simulink model "SetMultipleLedExample"  (R2015a)
settings: Solver=ode3  SolverMode=SingleTasking  StartTime=0.0  StopTime=10.0  RelTol=1e-3
settings Model: ExtModeTrigDuration=2  Creator=kkhoo  LastModifiedBy=kkhoo
settings OptimizationCC: OptimizeModelRefInitCode=on  LifeSpan=1
settings DebuggingCC: UnderspecifiedInitializationDetection=Classic  MergeDetectMultiDrivingBlocksExec=none
settings HardwareCC: ProdBitPerInt=16  ProdBitPerPointer=8  ProdIntDivRoundTo=Zero  ProdEndianess=LittleEndian  ProdWordSize=8  ProdHWDeviceType=Atmel->AVR
settings RTWCC: SystemTargetFile=realtime.tlc  GenerateMakefile=off  TemplateMakefile=realtime.tmf  Description=Run on Target Hardware  RTWVerbose=off
settings ERTTargetCC: CombineOutputUpdateFcns=off  ExtModeTransport=3  ExtModeMexFile=ext_serial_win32_comm_rtt  ExtModeMexArgs=0 1 9600  ERTSrcFileBannerTemplate=realtime_code_template.cgt  ERTHdrFileBannerTemplate=realtime_code_template.cgt  ERTDataSrcFileTemplate=realtime_code_template.cgt  ERTDataHdrFileTemplate=realtime_code_template.cgt  ERTCustomFileTemplate=realtime_file_process.tlc

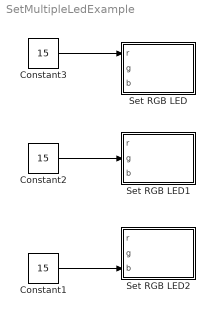
== system SetMultipleLedExample ==
  Constant1 : Constant  Value=15  OutDataTypeStr=Inherit: Inherit via back propagation
  Constant2 : Constant  Value=15  OutDataTypeStr=Inherit: Inherit via back propagation
  Constant3 : Constant  Value=15  OutDataTypeStr=Inherit: Inherit via back propagation
  Set RGB LED : MATLAB Function  LoadFcn=|  TreatAsAtomicUnit=on  mask(RGB LED){led_index=0}
      | set_param(gcs, 'CustomSource', strjoin(unique([strsplit(get_param(gcs, 'CustomSource')) ...
      |  'src/engduino_wrappers.cpp' 'src/Engduino.h'])));
      mask prompts: led_index "LED index"
      mask help:
      | Control the Red, Green and Blue color values of the LED specified by the LED index parameter.
      | Both the LED index and the three color values are of type uint8 and must be in the range 0-15.
      settings: AttributesFormatString=LED %<led_index>
  Set RGB LED1 : MATLAB Function  LoadFcn=|  TreatAsAtomicUnit=on  mask(RGB LED){led_index=1}
      | set_param(gcs, 'CustomSource', strjoin(unique([strsplit(get_param(gcs, 'CustomSource')) ...
      |  'src/engduino_wrappers.cpp' 'src/Engduino.h'])));
      mask prompts: led_index "LED index"
      mask help:
      | Control the Red, Green and Blue color values of the LED specified by the LED index parameter.
      | Both the LED index and the three color values are of type uint8 and must be in the range 0-15.
      settings: AttributesFormatString=LED %<led_index>
  Set RGB LED2 : MATLAB Function  LoadFcn=|  TreatAsAtomicUnit=on  mask(RGB LED){led_index=2}
      | set_param(gcs, 'CustomSource', strjoin(unique([strsplit(get_param(gcs, 'CustomSource')) ...
      |  'src/engduino_wrappers.cpp' 'src/Engduino.h'])));
      mask prompts: led_index "LED index"
      mask help:
      | Control the Red, Green and Blue color values of the LED specified by the LED index parameter.
      | Both the LED index and the three color values are of type uint8 and must be in the range 0-15.
      settings: AttributesFormatString=LED %<led_index>
  wires:
  Constant2/1 -> Set RGB LED1/2(g)
  Constant3/1 -> Set RGB LED/1(r)
  Constant1/1 -> Set RGB LED2/3(b)

== matlab function SetMultipleLedExample/Set RGB LED2 ==
  data: led_index parameter uint8 [0..15]; r input uint8 [0..15]; g input uint8 [0..15]; b input uint8 [0..15]
function rgb_led(led_index, r, g, b)

if strcmp(coder.target, 'rtw')
    coder.ceval('rgb_leds_wrapper', led_index, r, g, b);
end

== matlab function SetMultipleLedExample/Set RGB LED ==
  data: led_index parameter uint8 [0..15]; r input uint8 [0..15]; g input uint8 [0..15]; b input uint8 [0..15]
function rgb_led(led_index, r, g, b)

if strcmp(coder.target, 'rtw')
    coder.ceval('rgb_leds_wrapper', led_index, r, g, b);
end

== matlab function SetMultipleLedExample/Set RGB LED1 ==
  data: led_index parameter uint8 [0..15]; r input uint8 [0..15]; g input uint8 [0..15]; b input uint8 [0..15]
function rgb_led(led_index, r, g, b)

if strcmp(coder.target, 'rtw')
    coder.ceval('rgb_leds_wrapper', led_index, r, g, b);
end
